simulink model "untitled1"  (R2023a)
settings: Solver=VariableStepAuto  StartTime=0.0  StopTime=10.0  RelTol=1e-3
settings Model: Creator=BRL  LastModifiedBy=BRL

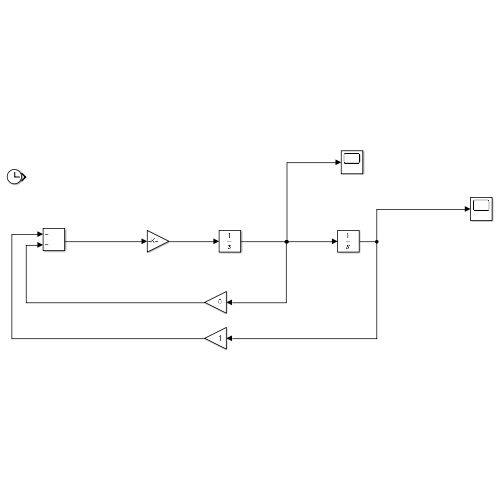
[thumbnail: Simulink's stored preview of the top-level diagram]
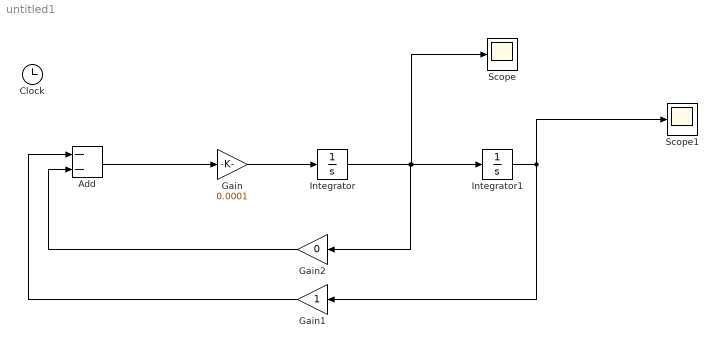
== system untitled1 ==
  Add : Sum  Inputs=--
  Clock : Clock
  Gain : Gain  Gain=0.0001
  Gain1 : Gain
  Gain2 : Gain  Gain=0
  Integrator : Integrator
  Integrator1 : Integrator  InitialCondition=100
  Scope : Scope
  Scope1 : Scope
  wires:
  Gain/1 -> Integrator/1
  Integrator/1 -> Gain2/1, Scope/1, Integrator1/1
  Integrator1/1 -> Scope1/1, Gain1/1
  Gain2/1 -> Add/2
  Gain1/1 -> Add/1
  Add/1 -> Gain/1
